simulink model "BLDCMotor"  (R2023a)
settings: Solver=VariableStepAuto  StartTime=0.0  StopTime=5  RelTol=1e-3
settings Model: Creator=raca  LastModifiedBy=headl
settings SolverCC: AlgebraicLoopSolver=TrustRegion
settings DataIOCC: ReturnWorkspaceOutputs=off
settings DebuggingCC: UnconnectedInputMsg=warning  UnconnectedOutputMsg=warning  UnconnectedLineMsg=warning  ArithmeticOperatorsInVariantConditions=warning
settings ModelReferenceCC: EnableRefExpFcnMdlSchedulingChecks=on
settings SFSimCC: SimUseLocalCustomCode=off  CustomCodeUndefinedFunction=UseInterfaceOnly
settings RTWCC: RTWUseLocalCustomCode=off
settings CodeAppCC: StateflowObjectComments=on

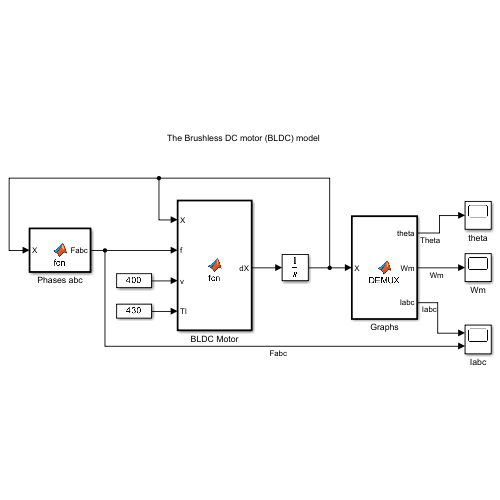
[thumbnail: Simulink's stored preview of the top-level diagram]
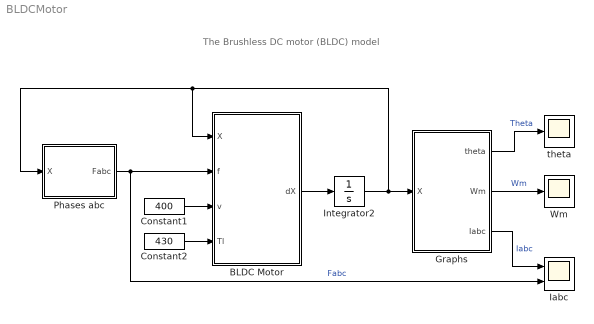
== system BLDCMotor ==
  note: The Brushless DC motor (BLDC) model
  BLDC Motor : MATLAB Function  TreatAsAtomicUnit=on
  Constant1 : Constant  Value=400
  Constant2 : Constant  Value=430
  Graphs : MATLAB Function  TreatAsAtomicUnit=on
  Iabc : Scope  NumInputPorts=2
  Integrator2 : Integrator  InitialCondition=[0;0;0;0.1;0]
  Phases abc : MATLAB Function  TreatAsAtomicUnit=on
  Wm : Scope
  theta : Scope
  wires:
  Graphs/1(theta) -> theta/1  "Theta"
  Integrator2/1 -> BLDC Motor/1(X), Phases abc/1(X), Graphs/1(X)
  BLDC Motor/1(dX) -> Integrator2/1
  Constant1/1 -> BLDC Motor/3(v)
  Constant2/1 -> BLDC Motor/4(Tl)
  Graphs/3(Iabc) -> Iabc/1  "Iabc"
  Phases abc/1(Fabc) -> Iabc/2, BLDC Motor/2(f)  "Fabc"
  Graphs/2(Wm) -> Wm/1  "Wm"

== matlab function BLDCMotor/BLDC Motor ==
  data: X input; f input; v input; dX output; Tl input
% L.Arturo Torres-Romero
% BLDC model

function dX = fcn(X,f,v,Tl)
u = [v.*f;Tl]; 
i_a = X(1); i_b = X(2); i_c = X(3); wm = X(4); theta = X(5);

R = 0.7;         %hase resistance.
L = 0.00383;     %Phase self-inductance.
M = 0.003;       %Phase Mutual inductance.
J = 0.6;         % Rotor inertia.
P = 4;           % Number of poles.
b = 0.0632177;   % Friction coefficient.
lambda = 0.9;    %is the Back EMF constant in v/rad/s.

A =[-(R/(L-M)) 0 0 -(lambda/(L-M))*f(1) 0;...
    0 -(R/(L-M)) 0 -(lambda/(L-M))*f(2) 0;...
    0 0 -(R/(L-M)) -(lambda/(L-M))*f(3) 0;...
    (lambda/J)*f(1) (lambda/J)*f(2) (lambda/J)*f(3) -b/J 0;...
    0 0 0 P/2 0];

B = diag([1/(L-M) 1/(L-M) 1/(L-M) -1/J]);
B = [B;0 0 0 0];

dX = A*X + B*u;   % model in the state-space

end

== matlab function BLDCMotor/Phases abc ==
  data: X input; Fabc output
% L.Arturo Torres-Romero
% BLDC trapezoidal shape functions

function Fabc = fcn(X)
Fabc = [0;0;0];
    theta = mod(X(5),2*pi);
    
    if (0<=theta)&&(theta<(pi/6))
        Fa = (6/pi)*theta;
    elseif ((pi/6)<=theta)&&(theta<(5*pi/6))
        Fa = 1;
    elseif ((5*pi/6<=theta))&&(theta<(7*pi/6))
        Fa = (6/pi)*(pi-theta);
    elseif ((7*pi/6)<=theta)&&(theta<(11*pi/6))
        Fa = -1;
    elseif ((11*pi/6)<=theta)&&(theta<(2*pi))
        Fa = (6/pi)*(theta-2*pi);
    else
        Fa = NaN;
    end
    
    if (0<=theta)&&(theta<(3*pi/6))
        Fb = -1;
    elseif ((3*pi/6)<=theta)&&(theta<(5*pi/6))
        Fb = (6/pi)*(theta-(2*pi)/3);
    elseif ((5*pi/6)<=theta)&&(theta<(9*pi/6))
        Fb = 1;
    elseif ((9*pi/6)<=theta)&&(theta<(11*pi/6))
        Fb = (6/pi)*(-theta+(5*pi)/3);
    elseif ((11*pi/6)<=theta)&&(theta<(2*pi))
        Fb = -1;
    else
        Fb = NaN;
    end
    
    if (0<=theta)&&(theta<(pi/6))
        Fc = 1;
    elseif ((pi/6)<=theta)&&(theta<(3*pi/6))
        Fc = (6/pi)*(pi/3-theta);
    elseif ((3*pi/6)<=theta)&&(theta<(7*pi/6))
        Fc = -1;
    elseif ((7*pi/6)<=theta)&&(theta<(9*pi/6))
        Fc = (6/pi)*(theta-(4*pi)/3);
    elseif ((9*pi/6)<=theta)&&(theta<(2*pi))
        Fc = 1;
    else
        Fc = NaN; 
    end
    
    Fabc = [Fa;Fb;Fc];
end

== matlab function BLDCMotor/Graphs ==
  data: X input; theta output; Wm output; Iabc output
function [theta,Wm,Iabc] = DEMUX(X)
theta = X(5); Wm = X(4);Iabc = X(1:3);
